simulink model "Control_SM_2022a"  (R2022a)
settings: configuration reference "Configuration_OBC6k6" (kept outside this file)
undefined symbols (not defined in the file): PFC_Vcmd_target, PFC_Vcmd_tolerance, sqrt_two
settings Model: DataDictionary=OBC6k6_DataStore.sldd  Creator=MartinChou  LastModifiedBy=LeoLai
settings ConfigSetRef: SourceName=Configuration_OBC6k6

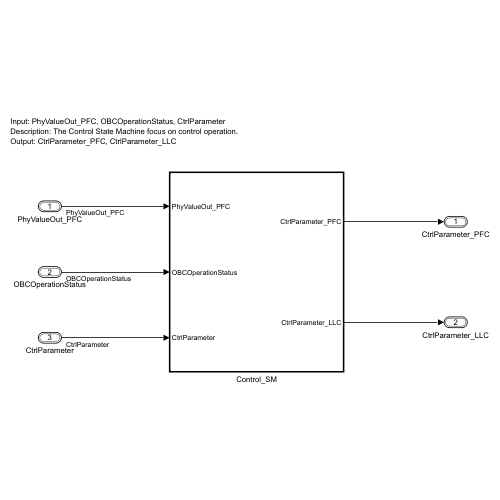
[thumbnail: Simulink's stored preview of the top-level diagram]
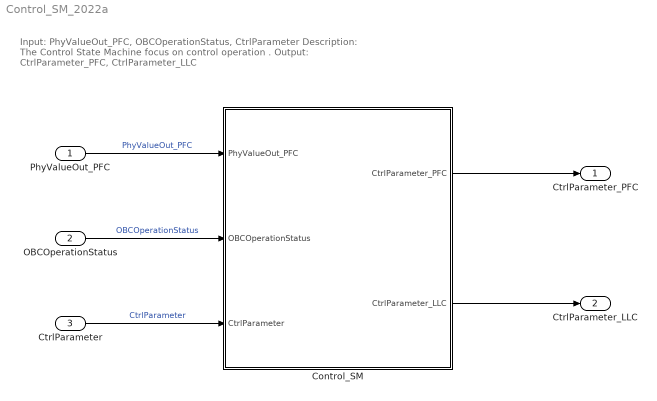
== system Control_SM_2022a ==
  note: Input: PhyValueOut_PFC, OBCOperationStatus, CtrlParameter
      | Description: The Control State Machine focus on control operation .
      | Output: CtrlParameter_PFC, CtrlParameter_LLC
  PhyValueOut_PFC : Inport  OutDataTypeStr=Bus: PhyValueOut_PFC_t
  OBCOperationStatus : Inport  Port=2  OutDataTypeStr=Bus: OBCOperationStatus_t
  CtrlParameter : Inport  Port=3  OutDataTypeStr=Bus: CtrlParameter_t
  Control_SM : Subsystem  TreatAsAtomicUnit=on
  CtrlParameter_PFC : Outport  OutDataTypeStr=Bus: CtrlParameter_PFC_t
  CtrlParameter_LLC : Outport  Port=2  OutDataTypeStr=Bus: CtrlParameter_LLC_t
  wires:
  PhyValueOut_PFC/1 -> Control_SM/1(PhyValueOut_PFC)  "PhyValueOut_PFC"
  Control_SM/2(CtrlParameter_LLC) -> CtrlParameter_LLC/1
  Control_SM/1(CtrlParameter_PFC) -> CtrlParameter_PFC/1
  CtrlParameter/1 -> Control_SM/3(CtrlParameter)  "CtrlParameter"
  OBCOperationStatus/1 -> Control_SM/2(OBCOperationStatus)  "OBCOperationStatus"

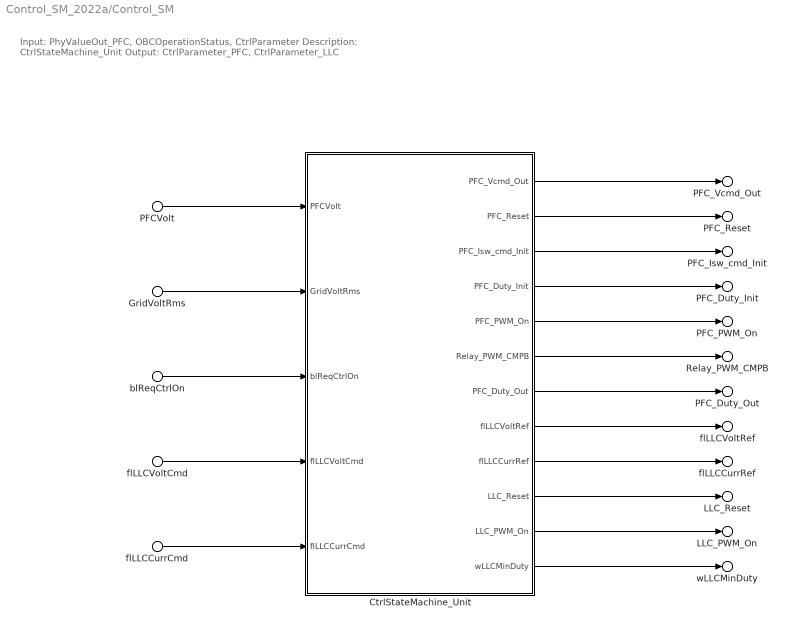
== system Control_SM_2022a/Control_SM ==
  note: Input: PhyValueOut_PFC, OBCOperationStatus, CtrlParameter
      | Description: CtrlStateMachine_Unit
      | Output: CtrlParameter_PFC, CtrlParameter_LLC
  GridVoltRms : Inport  PortName=PhyValueOut_PFC  Element=GridVoltRms
  PFCVolt : Inport  PortName=PhyValueOut_PFC  Element=PFCVolt
  blReqCtrlOn : Inport  Port=2  PortName=OBCOperationStatus  Element=blReqCtrlOn
  flLLCVoltCmd : Inport  Port=3  PortName=CtrlParameter  Element=flLLCVoltCmd
  flLLCCurrCmd : Inport  Port=3  PortName=CtrlParameter  Element=flLLCCurrCmd
  CtrlStateMachine_Unit : Subsystem
  PFC_Vcmd_Out : Outport  VectorParamsAs1DForOutWhenUnconnected=off  PortName=CtrlParameter_PFC  Element=PFC_Vcmd_Out
  PFC_Reset : Outport  VectorParamsAs1DForOutWhenUnconnected=off  PortName=CtrlParameter_PFC  Element=PFC_Reset
  PFC_Isw_cmd_Init : Outport  VectorParamsAs1DForOutWhenUnconnected=off  PortName=CtrlParameter_PFC  Element=PFC_Isw_cmd_Init
  PFC_Duty_Init : Outport  VectorParamsAs1DForOutWhenUnconnected=off  PortName=CtrlParameter_PFC  Element=PFC_Duty_Init
  PFC_PWM_On : Outport  VectorParamsAs1DForOutWhenUnconnected=off  PortName=CtrlParameter_PFC  Element=PFC_PWM_On
  Relay_PWM_CMPB : Outport  VectorParamsAs1DForOutWhenUnconnected=off  PortName=CtrlParameter_PFC  Element=Relay_PWM_CMPB
  PFC_Duty_Out : Outport  VectorParamsAs1DForOutWhenUnconnected=off  PortName=CtrlParameter_PFC  Element=PFC_Duty_Out
  flLLCVoltRef : Outport  Port=2  VectorParamsAs1DForOutWhenUnconnected=off  PortName=CtrlParameter_LLC  Element=flLLCVoltRef
  flLLCCurrRef : Outport  Port=2  VectorParamsAs1DForOutWhenUnconnected=off  PortName=CtrlParameter_LLC  Element=flLLCCurrRef
  LLC_Reset : Outport  Port=2  VectorParamsAs1DForOutWhenUnconnected=off  PortName=CtrlParameter_LLC  Element=LLC_Reset
  LLC_PWM_On : Outport  Port=2  VectorParamsAs1DForOutWhenUnconnected=off  PortName=CtrlParameter_LLC  Element=LLC_PWM_On
  wLLCMinDuty : Outport  Port=2  VectorParamsAs1DForOutWhenUnconnected=off  PortName=CtrlParameter_LLC  Element=wLLCMinDuty
  wires:
  PFCVolt/1 -> CtrlStateMachine_Unit/1(PFCVolt)
  GridVoltRms/1 -> CtrlStateMachine_Unit/2(GridVoltRms)
  blReqCtrlOn/1 -> CtrlStateMachine_Unit/3(blReqCtrlOn)
  flLLCVoltCmd/1 -> CtrlStateMachine_Unit/4(flLLCVoltCmd)
  flLLCCurrCmd/1 -> CtrlStateMachine_Unit/5(flLLCCurrCmd)
  CtrlStateMachine_Unit/1(PFC_Vcmd_Out) -> PFC_Vcmd_Out/1
  CtrlStateMachine_Unit/2(PFC_Reset) -> PFC_Reset/1
  CtrlStateMachine_Unit/3(PFC_Isw_cmd_Init) -> PFC_Isw_cmd_Init/1
  CtrlStateMachine_Unit/4(PFC_Duty_Init) -> PFC_Duty_Init/1
  CtrlStateMachine_Unit/5(PFC_PWM_On) -> PFC_PWM_On/1
  CtrlStateMachine_Unit/6(Relay_PWM_CMPB) -> Relay_PWM_CMPB/1
  CtrlStateMachine_Unit/7(PFC_Duty_Out) -> PFC_Duty_Out/1
  CtrlStateMachine_Unit/8(flLLCVoltRef) -> flLLCVoltRef/1
  CtrlStateMachine_Unit/9(flLLCCurrRef) -> flLLCCurrRef/1
  CtrlStateMachine_Unit/10(LLC_Reset) -> LLC_Reset/1
  CtrlStateMachine_Unit/11(LLC_PWM_On) -> LLC_PWM_On/1
  CtrlStateMachine_Unit/12(wLLCMinDuty) -> wLLCMinDuty/1

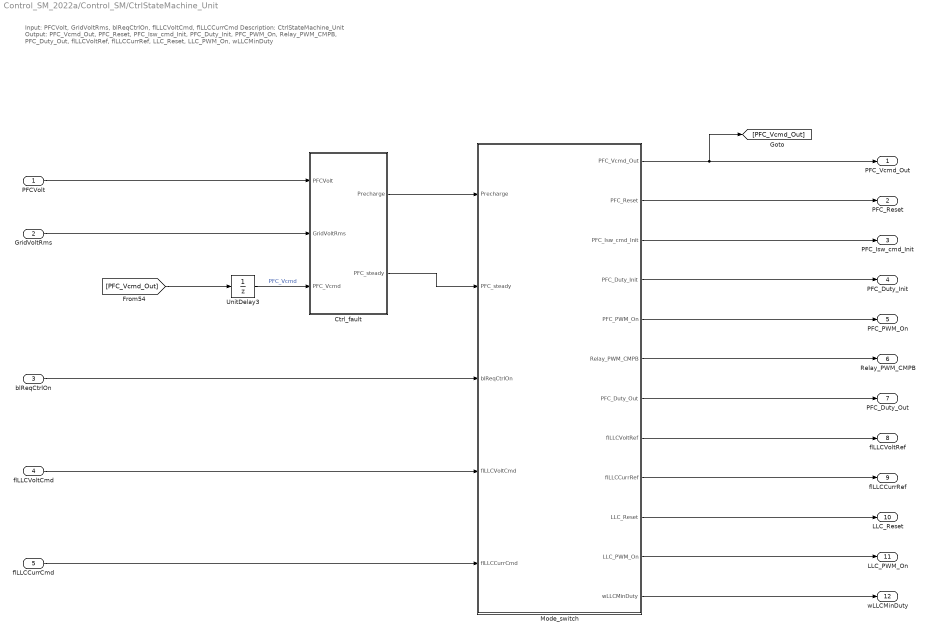
== system Control_SM_2022a/Control_SM/CtrlStateMachine_Unit ==
  note: Input: PFCVolt, GridVoltRms, blReqCtrlOn, flLLCVoltCmd, flLLCCurrCmd
      | Description: CtrlStateMachine_Unit
      | Output: PFC_Vcmd_Out, PFC_Reset, PFC_Isw_cmd_Init, PFC_Duty_Init, PFC_PWM_On, Relay_PWM_CMPB, PFC_Duty_Out, flLLCVoltRef, flLLCCurrRef, LLC_Reset, LLC_PWM_On, wLLCMinDuty
  PFCVolt : Inport
  GridVoltRms : Inport  Port=2
  blReqCtrlOn : Inport  Port=3
  flLLCVoltCmd : Inport  Port=4
  flLLCCurrCmd : Inport  Port=5
  Ctrl_fault : Subsystem
  Mode_switch : Subsystem
  UnitDelay3 : UnitDelay  SampleTime=-1  HasFrameUpgradeWarning=on
  PFC_Vcmd_Out : Outport
  PFC_Reset : Outport  Port=2
  PFC_Isw_cmd_Init : Outport  Port=3
  PFC_Duty_Init : Outport  Port=4
  PFC_PWM_On : Outport  Port=5
  Relay_PWM_CMPB : Outport  Port=6
  PFC_Duty_Out : Outport  Port=7
  flLLCVoltRef : Outport  Port=8
  flLLCCurrRef : Outport  Port=9
  LLC_Reset : Outport  Port=10
  LLC_PWM_On : Outport  Port=11
  wLLCMinDuty : Outport  Port=12
  wires:
  Mode_switch/1(PFC_Vcmd_Out) -> PFC_Vcmd_Out/1, [PFC_Vcmd_Out]
  Mode_switch/11(LLC_PWM_On) -> LLC_PWM_On/1
  Ctrl_fault/1(Precharge) -> Mode_switch/1(Precharge)
  Mode_switch/10(LLC_Reset) -> LLC_Reset/1
  [PFC_Vcmd_Out] -> UnitDelay3/1
  UnitDelay3/1 -> Ctrl_fault/3(PFC_Vcmd)  "PFC_Vcmd"
  GridVoltRms/1 -> Ctrl_fault/2(GridVoltRms)
  Ctrl_fault/2(PFC_steady) -> Mode_switch/2(PFC_steady)
  flLLCVoltCmd/1 -> Mode_switch/4(flLLCVoltCmd)
  Mode_switch/8(flLLCVoltRef) -> flLLCVoltRef/1
  blReqCtrlOn/1 -> Mode_switch/3(blReqCtrlOn)
  flLLCCurrCmd/1 -> Mode_switch/5(flLLCCurrCmd)
  Mode_switch/9(flLLCCurrRef) -> flLLCCurrRef/1
  Mode_switch/12(wLLCMinDuty) -> wLLCMinDuty/1
  Mode_switch/7(PFC_Duty_Out) -> PFC_Duty_Out/1
  Mode_switch/2(PFC_Reset) -> PFC_Reset/1
  Mode_switch/3(PFC_Isw_cmd_Init) -> PFC_Isw_cmd_Init/1
  Mode_switch/5(PFC_PWM_On) -> PFC_PWM_On/1
  Mode_switch/6(Relay_PWM_CMPB) -> Relay_PWM_CMPB/1
  PFCVolt/1 -> Ctrl_fault/1(PFCVolt)
  Mode_switch/4(PFC_Duty_Init) -> PFC_Duty_Init/1

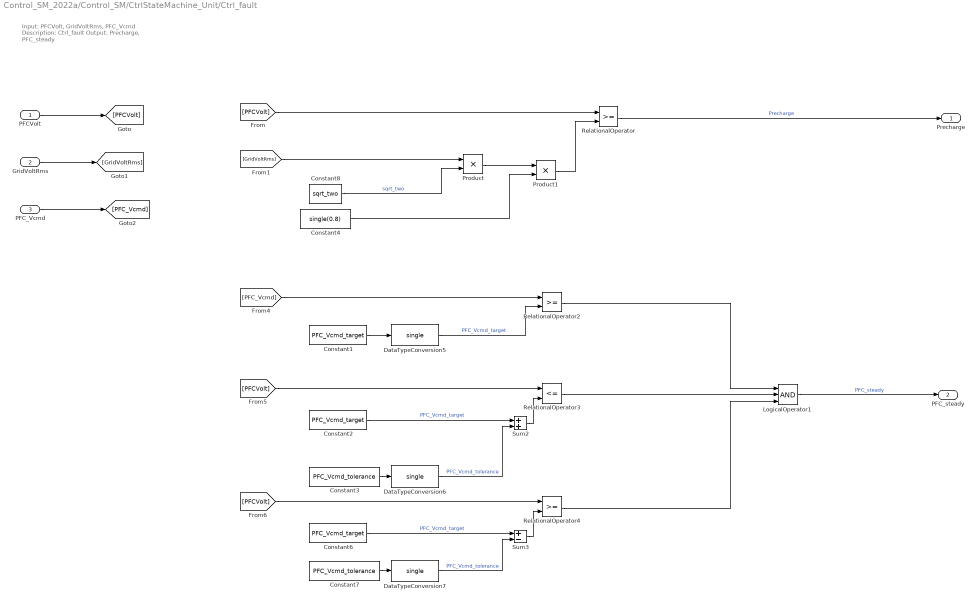
== system Control_SM_2022a/Control_SM/CtrlStateMachine_Unit/Ctrl_fault ==
  note: Input: PFCVolt, GridVoltRms, PFC_Vcmd
      | Description: Ctrl_fault
      | Output: Precharge, PFC_steady
  PFCVolt : Inport
  GridVoltRms : Inport  Port=2
  PFC_Vcmd : Inport  Port=3
  Constant1 : Constant  Value=PFC_Vcmd_target
  Constant2 : Constant  Value=PFC_Vcmd_target
  Constant3 : Constant  Value=PFC_Vcmd_tolerance
  Constant4 : Constant  Value=single(0.8)
  Constant6 : Constant  Value=PFC_Vcmd_target
  Constant7 : Constant  Value=PFC_Vcmd_tolerance
  Constant8 : Constant  Value=sqrt_two
  DataTypeConversion5 : DataTypeConversion  OutDataTypeStr=single  SaturateOnIntegerOverflow=off  RndMeth=Floor
  DataTypeConversion6 : DataTypeConversion  OutDataTypeStr=single  SaturateOnIntegerOverflow=off  RndMeth=Floor
  DataTypeConversion7 : DataTypeConversion  OutDataTypeStr=single  SaturateOnIntegerOverflow=off  RndMeth=Floor
  LogicalOperator1 : Logic  Inputs=3  AllPortsSameDT=off
  Product : Product
  Product1 : Product
  RelationalOperator : RelationalOperator  RndMeth=Simplest  InputSameDT=off
  RelationalOperator2 : RelationalOperator  RndMeth=Simplest  InputSameDT=off
  RelationalOperator3 : RelationalOperator  Operator=<=  RndMeth=Simplest  InputSameDT=off
  RelationalOperator4 : RelationalOperator  RndMeth=Simplest  InputSameDT=off
  Sum2 : Sum
  Sum3 : Sum  Inputs=+-
  Precharge : Outport
  PFC_steady : Outport  Port=2
  wires:
  [GridVoltRms] -> Product/1
  Product1/1 -> RelationalOperator/2
  Constant4/1 -> Product1/2
  Product/1 -> Product1/1
  [PFCVolt] -> RelationalOperator/1
  PFCVolt/1 -> [PFCVolt]
  GridVoltRms/1 -> [GridVoltRms]
  PFC_Vcmd/1 -> [PFC_Vcmd]
  [PFC_Vcmd] -> RelationalOperator2/1
  Constant1/1 -> DataTypeConversion5/1
  [PFCVolt] -> RelationalOperator3/1
  Constant2/1 -> Sum2/1  "PFC_Vcmd_target"
  Sum2/1 -> RelationalOperator3/2
  Constant3/1 -> DataTypeConversion6/1
  Constant7/1 -> DataTypeConversion7/1
  Sum3/1 -> RelationalOperator4/2
  Constant6/1 -> Sum3/1  "PFC_Vcmd_target"
  [PFCVolt] -> RelationalOperator4/1
  Constant8/1 -> Product/2  "sqrt_two"
  LogicalOperator1/1 -> PFC_steady/1  "PFC_steady"
  RelationalOperator/1 -> Precharge/1  "Precharge"
  RelationalOperator2/1 -> LogicalOperator1/1
  RelationalOperator3/1 -> LogicalOperator1/2
  RelationalOperator4/1 -> LogicalOperator1/3
  DataTypeConversion5/1 -> RelationalOperator2/2  "PFC_Vcmd_target"
  DataTypeConversion6/1 -> Sum2/2  "PFC_Vcmd_tolerance"
  DataTypeConversion7/1 -> Sum3/2  "PFC_Vcmd_tolerance"

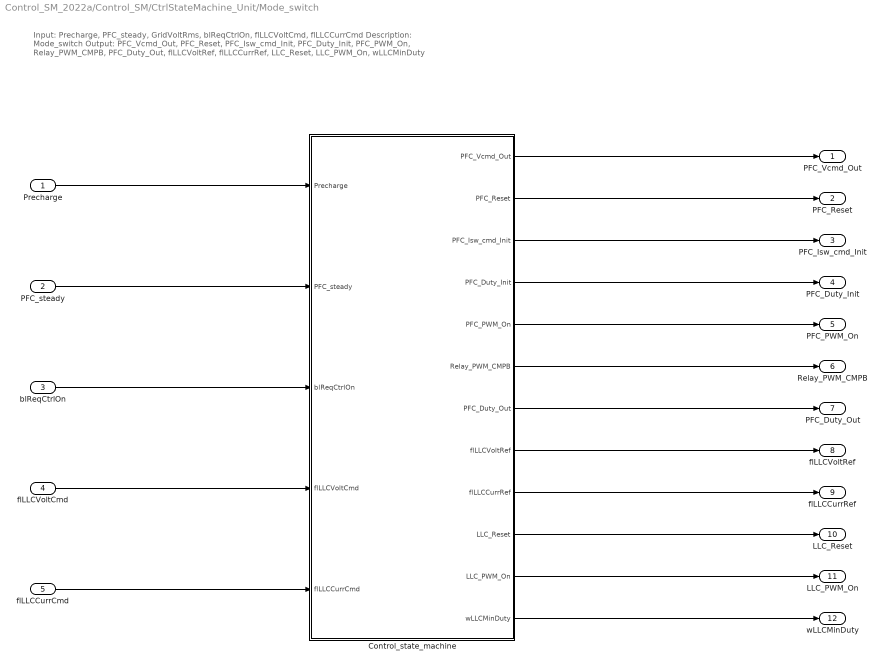
== system Control_SM_2022a/Control_SM/CtrlStateMachine_Unit/Mode_switch ==
  note: Input: Precharge, PFC_steady, GridVoltRms, blReqCtrlOn, flLLCVoltCmd, flLLCCurrCmd
      | Description: Mode_switch
      | Output: PFC_Vcmd_Out, PFC_Reset, PFC_Isw_cmd_Init, PFC_Duty_Init, PFC_PWM_On, Relay_PWM_CMPB, PFC_Duty_Out, flLLCVoltRef, flLLCCurrRef, LLC_Reset, LLC_PWM_On, wLLCMinDuty
  Precharge : Inport
  PFC_steady : Inport  Port=2
  blReqCtrlOn : Inport  Port=3
  flLLCVoltCmd : Inport  Port=4
  flLLCCurrCmd : Inport  Port=5
  Control_state_machine : Stateflow chart  TreatAsAtomicUnit=on
      settings: PortSchema="{\"entries\":[{\"content\":{\"sides\":[{\"content\":{\"connectorIds\":[\"In1\",\"In2\",\"In3\",\"In4\",\"In5\"]},\"type\":\"ConnectorPlacement.EquallySpacedRectSide\",\"uuid\":\"64cd7549-e4a6-4907-902e-b2fde3590740\"},{\"content\":{\"connectorIds\":[\"Out1\",\"Out2\",\"Out3\",\"Out4\",\"Out8\",\"Out10\",\"Out12\",\"Out5\",\"Out7\",\"Out6\",\"Out9\",\"Out11\"],\"side\":\"RIGHT\"},\"type\":\"ConnectorPlacement.EquallySpacedRectSide\",\"uuid\":\"de1e121e-478a-4bb0-95d7-9652cb54a65b\"},{\"content\":{\"connectorIds\":[],\"side\":\"TOP\"},\"type\":\"ConnectorPlacement.EquallySpacedRectSide\",\"uuid\":\"0de0764e-4e9b-40be-82ac-42b7f51d04bc\"}]},\"type\":\"ConnectorPlacement.EquallySpacedConnector\",\"uuid\":\"973ffa16-2269-456b-9131-027f1e2169ff\"}],\"packageUris\":[\"http://schema.mathworks.com/mf0/Connector/R2020b\"],\"version\":\"1.0\"}"
  PFC_Vcmd_Out : Outport
  PFC_Reset : Outport  Port=2
  PFC_Isw_cmd_Init : Outport  Port=3
  PFC_Duty_Init : Outport  Port=4
  PFC_PWM_On : Outport  Port=5
  Relay_PWM_CMPB : Outport  Port=6
  PFC_Duty_Out : Outport  Port=7
  flLLCVoltRef : Outport  Port=8
  flLLCCurrRef : Outport  Port=9
  LLC_Reset : Outport  Port=10
  LLC_PWM_On : Outport  Port=11
  wLLCMinDuty : Outport  Port=12
  wires:
  flLLCCurrCmd/1 -> Control_state_machine/5(flLLCCurrCmd)
  Precharge/1 -> Control_state_machine/1(Precharge)
  Control_state_machine/2(PFC_Reset) -> PFC_Reset/1
  PFC_steady/1 -> Control_state_machine/2(PFC_steady)
  flLLCVoltCmd/1 -> Control_state_machine/4(flLLCVoltCmd)
  blReqCtrlOn/1 -> Control_state_machine/3(blReqCtrlOn)
  Control_state_machine/3(PFC_Isw_cmd_Init) -> PFC_Isw_cmd_Init/1
  Control_state_machine/4(PFC_Duty_Init) -> PFC_Duty_Init/1
  Control_state_machine/6(LLC_Reset) -> LLC_Reset/1
  Control_state_machine/8(PFC_PWM_On) -> PFC_PWM_On/1
  Control_state_machine/9(LLC_PWM_On) -> LLC_PWM_On/1
  Control_state_machine/1(PFC_Vcmd_Out) -> PFC_Vcmd_Out/1
  Control_state_machine/5(flLLCVoltRef) -> flLLCVoltRef/1
  Control_state_machine/7(flLLCCurrRef) -> flLLCCurrRef/1
  Control_state_machine/10(Relay_PWM_CMPB) -> Relay_PWM_CMPB/1
  Control_state_machine/11(wLLCMinDuty) -> wLLCMinDuty/1
  Control_state_machine/12(PFC_Duty_Out) -> PFC_Duty_Out/1

== stateflow chart Control_SM_2022a/Control_SM/CtrlStateMachine_Unit/Mode_switch/Control_state_machine ==
  settings: updateMethod=DISCRETE
  state Reset
    PFC_PWM_On=false;
    LLC_PWM_On=false;
    PFC_Isw_cmd_Init=single(0);
    PFC_Duty_Init=single(0);
    PFC_Reset=true;
    LLC_Reset=true;
    Relay_PWM_CMPB = single(0);
    PFC_Vcmd_Out = single(100);
    flLLCVoltRef = single(0);
    flLLCCurrRef = single(0);
    wLLCMinDuty = uint16(330);
  state Duty_Softstart(PFC_Dutycmd, PFC_Dutyref) [function]
    (default) -> (junction 532)
    (junction 532) -> (junction 533) [order 1] : [PFC_Dutycmd < PFC_Dutyref]
    (junction 532) -> (junction 534) [order 2] : {
        |   PFC_DutyTemp = PFC_Dutyref;
        | }
    (junction 533) -> (junction 535) : {
        |   PFC_DutyTemp=PFC_Dutycmd+PFC_Dutysoft;
        | }
    (junction 535) -> (junction 534)
    (junction 534) -> (junction 536) : {
        |   PFC_Duty_Out = PFC_DutyTemp;
        | }
  state Action
    state Bulk_Precharge
      state Precharge_Check
        during:
        PFC_PWM_On = false;
        LLC_PWM_On = false;
        PFC_Reset = true;
        LLC_Reset = true;
        Relay_PWM_CMPB = single(0);
        flLLCVoltRef = single(0);
        flLLCCurrRef = single(0);
        wLLCMinDuty = uint16(330);
      state Relay_On
        during:
        PFC_PWM_On = false;
        LLC_PWM_On = false;
        PFC_Reset = true;
        LLC_Reset = true;
        Relay_PWM_CMPB = single(2600);
        flLLCVoltRef = single(0);
        flLLCCurrRef = single(0);
        wLLCMinDuty = uint16(330);
      state Waitting
        during:
        PFC_PWM_On = false;
        LLC_PWM_On = false;
        PFC_Reset= true;
        LLC_Reset = true;
        Relay_PWM_CMPB = single(0);
        flLLCVoltRef = single(0);
        flLLCCurrRef = single(0);
        wLLCMinDuty = uint16(330);
      (default) -> Precharge_Check
      Precharge_Check -> Waitting : [Precharge]
      Waitting -> Relay_On : after(10000, tick)
    state Bulk_Voltage_Establish
      state PFC_On
        during:
        PFC_PWM_On = true;
        LLC_PWM_On = false;
        PFC_Reset = false;
        LLC_Reset = true;
        Relay_PWM_CMPB = single(2600);
        PFC_Softstart(PFC_Vcmd_Out, 400);
        Duty_Softstart(PFC_Duty_Out, 1);
        flLLCVoltRef = single(0);
        flLLCCurrRef = single(0);
        wLLCMinDuty = uint16(330);
      state Bulk_Voltage_Check
        during:
        PFC_PWM_On = true;
        LLC_PWM_On = false;
        PFC_Reset = false;
        LLC_Reset = true;
        Relay_PWM_CMPB = single(1250);
        PFC_Softstart(PFC_Vcmd_Out, 400);
        flLLCVoltRef = single(0);
        flLLCCurrRef = single(0);
        wLLCMinDuty = uint16(330);
      (default) -> PFC_On
      PFC_On -> Bulk_Voltage_Check : after(19600, tick)
    state OBC_Output
      state OBC_SoftStart
        during:
        PFC_PWM_On = true;
        LLC_PWM_On = true;
        PFC_Reset = false;
        LLC_Reset = false;
        Relay_PWM_CMPB = single(1250);
        flLLCVoltRef = flLLCVoltRef + flVoltSoft;
        flLLCCurrRef = single(1);
        wLLCMinDuty = uint16(330);
      state OBC_Run
        during:
        PFC_PWM_On = true;
        LLC_PWM_On = true;
        LLC_Reset = false;
        Relay_PWM_CMPB = single(1250);
        flLLCVoltRef = flLLCVoltCmd;
        flLLCCurrRef = SoftStart(flLLCCurrRef, flLLCCurrCmd, flCurrSoft);
        wLLCMinDuty = uint16(417);
      (default) -> OBC_SoftStart
      OBC_SoftStart -> OBC_Run : [flLLCVoltRef >= flLLCVoltCmd]
    (default) -> Bulk_Precharge
    Relay_On -> Bulk_Voltage_Establish : after(400, tick)
    Bulk_Voltage_Check -> OBC_Output : after(8000, tick)[PFC_steady]
  state PFC_Softstart(PFC_Vcmd, PFC_Vref) [function]
    (default) -> (junction 336)
    (junction 336) -> (junction 340) [order 1] : [PFC_Vcmd < PFC_Vref]
    (junction 336) -> (junction 337) [order 2] : {
        |   PFC_Temp = PFC_Vref;
        | }
    (junction 340) -> (junction 341) : {
        |   PFC_Temp=PFC_Vcmd+PFC_Vsoft;
        | }
    (junction 341) -> (junction 337)
    (junction 337) -> (junction 339) : {
        |   PFC_Vcmd_Out = PFC_Temp;
        | }
  state flRefOut = SoftStart(flRef,flCmd, flSoftValue) [function]
    (default) -> (junction 501)
    (junction 501) -> (junction 519) [order 2] : [flRef > flCmd]
    (junction 501) -> (junction 507) [order 1] : [flRef < flCmd]
    (junction 519) -> (junction 521) : {
        |   flRef = flRef - flSoftValue;
        | }
    (junction 501) -> (junction 510) [order 3] : {
        |   flRef = flCmd;
        | }
    (junction 507) -> (junction 509) : {
        |   flRef = flRef + flSoftValue;
        | }
    (junction 521) -> (junction 510)
    (junction 509) -> (junction 510)
    (junction 510) -> (junction 511) : {
        | flRefOut = flRef
        | }
  (default) -> Reset
  Bulk_Precharge -> Reset : after(200000, tick)[!Precharge]
  Action -> Reset : [!blReqCtrlOn]
  Reset -> Action : [blReqCtrlOn]
  data: PFC_Dutycmd function_input single; PFC_Dutyref function_input single; PFC_Vcmd function_input single; PFC_Vref function_input single; flRef function_input single; flCmd function_input single; flSoftValue function_input single; flRefOut function_output single; PFC_Vcmd_Out output single =100; PFC_Reset output boolean; PFC_Isw_cmd_Init output single; PFC_Duty_Init output single; flLLCVoltRef output single =0; LLC_Reset output boolean; flLLCCurrRef output single =0; Precharge input boolean; PFC_steady input boolean; blReqCtrlOn input boolean; PFC_PWM_On output boolean; LLC_PWM_On output boolean; flCurrSoft local single =0.00025; flVoltSoft local single =0.1; PFC_Vsoft local single =0.03; PFC_Temp local single =0; flLLCVoltCmd input single; flLLCCurrCmd input single; Relay_PWM_CMPB output single; wLLCMinDuty output uint16; PFC_Duty_Out output single =0.3; PFC_Dutysoft local single =0.0001; PFC_DutyTemp local single
